simulink model "PTSSE_SetData"  (R2016b)
settings: configuration reference "CodeGenConfigSet" (kept outside this file)
undefined symbols (not defined in the file or in its folder): PT_TraType_State_conv
settings Model: Creator=Wollf  LastModifiedBy=Wollf
settings ConfigSetRef: SourceLocation=Base Workspace

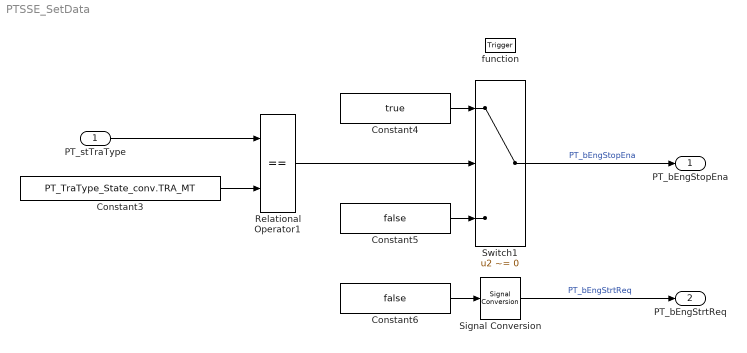
== system PTSSE_SetData ==
  PT_stTraType : Inport  Description=Current transmission type  OutDataTypeStr=Enum: PT_TraType_State_conv
  function : TriggerPort  TriggerType=function-call  VariantControl=Variant
  Constant3 : Constant  Value=PT_TraType_State_conv.TRA_MT
  Constant4 : Constant  Value=true  OutDataTypeStr=boolean
  Constant5 : Constant  Value=false  OutDataTypeStr=boolean
  Constant6 : Constant  Value=false  OutDataTypeStr=boolean
  Relational Operator1 : RelationalOperator  Operator===  OutDataTypeStr=boolean  RndMeth=Simplest  InputSameDT=on
  Signal Conversion : SignalConversion  OverrideOpt=off
  Switch1 : Switch  Criteria=u2 ~= 0  InputSameDT=on
  PT_bEngStopEna : Outport  Description=Engine stop request of transmission  OutMin=0  OutMax=1  OutDataTypeStr=boolean
  PT_bEngStrtReq : Outport  Description=Engine start request of transmission  Port=2  OutMin=0  OutMax=1  OutDataTypeStr=boolean
  wires:
  Constant4/1 -> Switch1/1
  Relational Operator1/1 -> Switch1/2
  Switch1/1 -> PT_bEngStopEna/1  "PT_bEngStopEna"
  PT_stTraType/1 -> Relational Operator1/1
  Constant3/1 -> Relational Operator1/2
  Constant5/1 -> Switch1/3
  Constant6/1 -> Signal Conversion/1
  Signal Conversion/1 -> PT_bEngStrtReq/1  "PT_bEngStrtReq"
